simulink model "controller"  (R2020b)
settings: Solver=VariableStepAuto  StartTime=0.0  StopTime=10.0  RelTol=1e-3
libraries: roblocks x3
settings Model: Creator=yrza  LastModifiedBy=аааа

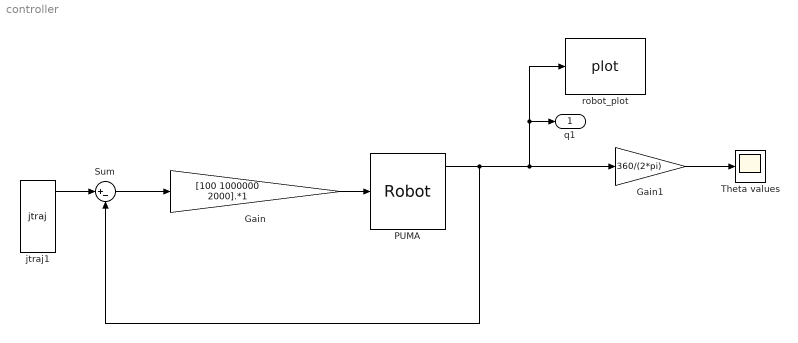
== system controller ==
  Gain : Gain  Gain=[100 1000000 2000].*1
  Gain1 : Gain  Gain=360/(2*pi)
  PUMA : roblocks/Arm/Robot  robot=rrr  q0=[0 0 0]
  Sum : Sum  Inputs=|+-
  Theta values : Scope
  jtraj1 : roblocks/Toolbox/jtraj  q0=[0 0 0]  qf=[pi/2 -pi/4 -pi/4]  tmax=2  ts=0.02
  robot_plot : roblocks/Arm/plot  robot=rrr  fps=5  holdplot=on
  q1 : Outport
  wires:
  PUMA/1 -> robot_plot/1, q1/1, Gain1/1, Sum/2
  Gain/1 -> PUMA/1
  Gain1/1 -> Theta values/1
  Sum/1 -> Gain/1
  jtraj1/1 -> Sum/1
